simulink model "gazeboExamplePerceptionCustom"  (R2017b)
settings: Solver=FixedStepDiscrete  StartTime=0.0  StopTime=inf  FixedStep=perceptionTs  RelTol=1e-3  EnableMultiTasking=on
PreLoadFcn:
  | params = controlParamsGazebo;
  | 
  | % Algorithm sample time
  | perceptionTs = 0.5;
  | 
  | rosshutdown;
  | loadIpAddresses;
  | rosinit(gazeboIp);
model workspace (MAT data in the model file):
  SL_ROS_VariableLengthArrays_MaxSizes.CommonInfo.ArrayTruncateAction = 'EmitWarning'
  SL_ROS_VariableLengthArrays_MaxSizes.MsgTypeMap = containers.Map
  SL_ROS_VariableLengthArrays_MaxSizes.MsgTypeMap.serialization.keys = {'sensor_msgs/Image'}
  SL_ROS_VariableLengthArrays_MaxSizes.MsgTypeMap.serialization.values{1}(1).PropertyName = 'Data'
  SL_ROS_VariableLengthArrays_MaxSizes.MsgTypeMap.serialization.values{1}(1).DataType = 'uint8'
  SL_ROS_VariableLengthArrays_MaxSizes.MsgTypeMap.serialization.values{1}(1).MaxLength = 921600
  SL_ROS_VariableLengthArrays_MaxSizes.MsgTypeMap.serialization.values{1}(2).PropertyName = 'Encoding'
  SL_ROS_VariableLengthArrays_MaxSizes.MsgTypeMap.serialization.values{1}(2).DataType = 'uint8'
  SL_ROS_VariableLengthArrays_MaxSizes.MsgTypeMap.serialization.values{1}(2).MaxLength = 128
  SL_ROS_VariableLengthArrays_MaxSizes.MsgTypeMap.serialization.uniformity = 0
  SL_ROS_VariableLengthArrays_MaxSizes.MsgTypeMap.serialization.keyType = 'char'
  SL_ROS_VariableLengthArrays_MaxSizes.MsgTypeMap.serialization.valueType = 'any'
undefined symbols (not defined in the file): BlobSize, CircleX, CircleY, ImgWidth
libraries: robotlib x4
settings Model: Creator=scastro  LastModifiedBy=scastro
settings SolverCC: PositivePriorityOrder=on
settings OptimizationCC: PassReuseOutputArgsAs=Individual arguments  MaxStackSize=64
settings DebuggingCC: ParameterTunabilityLossMsg=error
settings HardwareCC: ProdBitPerLong=64  ProdHWDeviceType=Intel->x86-64 (Linux 64)
settings RTWCC: SystemTargetFile=ert.tlc  HardwareBoard=Robot Operating System (ROS)  TemplateMakefile=ert_default_tmf  GenerateReport=on  Toolchain=Catkin  IncludeHyperlinkInReport=on  LaunchReport=on  TargetLang=C++  GenerateTraceInfo=on  GenerateTraceReport=on  GenerateTraceReportSl=on  GenerateTraceReportSf=on  GenerateTraceReportEml=on
settings CodeAppCC: ForceParamTrailComments=on  IgnoreCustomStorageClasses=off  OperatorAnnotations=on  SimulinkDataObjDesc=on  SFDataObjDesc=on  MATLABFcnDesc=on  InsertBlockDesc=on  StateflowObjectComments=on  MATLABSourceComments=on
settings ERTTargetCC: SupportVariableSizeSignals=on

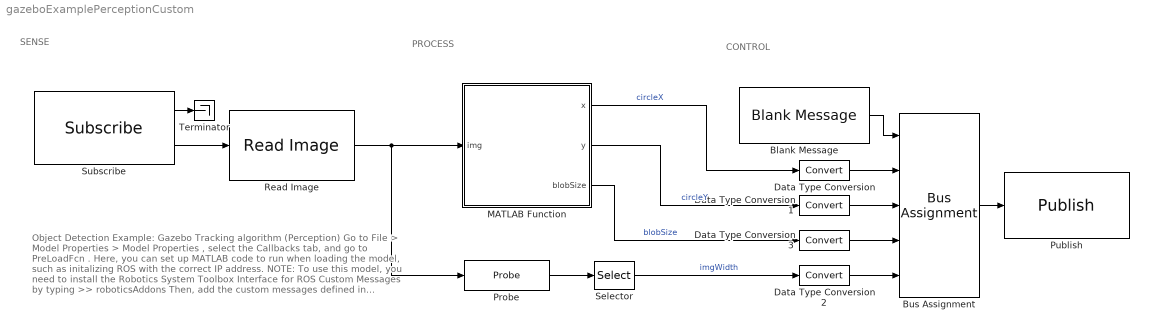
== system gazeboExamplePerceptionCustom ==
  note: CONTROL
  note: PROCESS
  note: SENSE
  note: Object Detection Example:
      | Gazebo Tracking algorithm (Perception)
      |
      | Go to File > Model Properties > Model Properties , select the Callbacks tab, and go to PreLoadFcn . Here, you can set up MATLAB code to run when loading the model, such as initalizing ROS with the correct IP address.
      |
      | NOTE: To use this model, you need to install the Robotics System Toolbox Interface for ROS Custom Messages by typing >> roboticsAddons
      | Then, add the custom messages defined in demoFiles/distributed/custom_robot_msgs
      |
      | Copyright 2017 The MathWorks, Inc.
  Blank Message : robotlib/Blank Message  SourceLibraryInfo=This block requires Robotics System Toolbox  messageType=custom_robot_msgs/circle_detection  SampleTime=inf
      settings: SourceProductBaseCode=RO
  Bus Assignment : BusAssignment  AssignedSignals=CircleX,CircleY,BlobSize,ImgWidth
  Data Type Conversion{,1..3} (4 alike) : DataTypeConversion
  MATLAB Function : MATLAB Function  TreatAsAtomicUnit=on
  Probe : Probe  ProbeWidth=off  ProbeSampleTime=off  ProbeComplexSignal=off  ProbeSignalDimensions=on
  Publish : robotlib/Publish  SourceLibraryInfo=This block requires Robotics System Toolbox  topicSource=Specify your own  topic=/ctrl_inputs  messageType=custom_robot_msgs/circle_detection  messageQueueLength=1
      settings: SourceProductBaseCode=RO
  Read Image : robotlib/Read Image  SourceLibraryInfo=This block requires Robotics System Toolbox  MaximumImageSize=[480, 640]  ImageEncoding=rgb8  ShowAlphaOutput=off  ShowErrorCodeOutput=off  VariableSizeOutputs=off
      settings: SourceProductName=Robotics System Toolbox  SourceProductBaseCode=RO
  Selector : Selector  InputPortWidth=3  IndexOptions=Index vector (dialog)  Indices=2  OutputSizes=1
  Subscribe : robotlib/Subscribe  SourceLibraryInfo=This block requires Robotics System Toolbox  topicSource=Select from ROS network  topic=/camera/rgb/image_raw  messageType=sensor_msgs/Image  sampleTime=-1  messageQueueLength=1
      settings: SourceProductBaseCode=RO
  Terminator : Terminator
  wires:
  MATLAB Function/1(x) -> Data Type Conversion/1  "circleX"
  Probe/1 -> Selector/1
  Subscribe/2 -> Read Image/1
  Read Image/1 -> MATLAB Function/1(img), Probe/1
  Subscribe/1 -> Terminator/1
  Bus Assignment/1 -> Publish/1
  Data Type Conversion2/1 -> Bus Assignment/5
  Data Type Conversion1/1 -> Bus Assignment/3
  Blank Message/1 -> Bus Assignment/1
  Selector/1 -> Data Type Conversion2/1  "imgWidth"
  MATLAB Function/3(blobSize) -> Data Type Conversion3/1  "blobSize"
  Data Type Conversion/1 -> Bus Assignment/2
  MATLAB Function/2(y) -> Data Type Conversion1/1  "circleY"
  Data Type Conversion3/1 -> Bus Assignment/4

== matlab function gazeboExamplePerceptionCustom/MATLAB Function ==
  data: x output; img input; y output; blobSize output
function [x,y,blobSize] = CircleDetection(img)
    
    % Initialize outputs
    x = 0;
    y = 0;
    blobSize = 0;
    
    % Call external function
    resizeScale = 0.5;
    [x,y,blobSize] = detectCircle(img,resizeScale);

end
